simulink model "MSFartoystyring"  (R2016a)
settings: Solver=ode45  StartTime=tstart  StopTime=tstop  RelTol=1e-3
values from neighbouring files (symbols this model uses):
  c = 0    [run_task_2_2.m]
  d1 = 1.0163    [run_task_2_2.m]
  d2 = 2.4413e-05    [run_task_2_2.m]
  K_d = (2*zeta*w_n*T - 1)/K    (= 268.173334927)    [run_task_2_2.m]
  K_i = K_p*w_n/10    (= 0.176946727827)    [run_task_2_2.m]
  K_is = lambda^2    [run_task_2_2.m]
  K_p = w_n^2*T/K    (= 17.6946727827)    [run_task_2_2.m]
  K_ps = 2*lambda    [run_task_2_2.m]
  m = 365.2560    (= 365.256)    [run_task_2_2.m]
  psi0 = deg2rad(150)    [run_task_2_2.m]
  r0 = 0    [run_task_2_2.m]
  tsamp = 10    [run_task_2_2.m]
  v0 = [6.63 0]'    [run_task_2_2.m]
  w_n = 0.1    [run_task_2_2.m]
  w_ns = 0.01    [run_task_2_2.m]
  zeta = 0.8    [run_task_2_2.m]
  zeta_s = 1    [run_task_2_2.m]
undefined symbols (not defined in the file or in its folder): msfartoystyring, WP
undefined symbols (not defined in the file): p0
settings Model: ExtModeAutoUpdateStatusClock=off  Creator=christh  LastModifiedBy=fredr
settings DataIOCC: LimitDataPoints=on  SaveFormat=Array  SignalLoggingSaveFormat=ModelDataLogs
settings OptimizationCC: ExpressionDepthLimit=2147483647  InitFltsAndDblsToZero=on
settings DebuggingCC: UnderspecifiedInitializationDetection=Classic  MergeDetectMultiDrivingBlocksExec=none  SolverPrmCheckMsg=warning  FcnCallInpInsideContextMsg=UseLocalSettings  AllowSymbolicDim=off  StateNameClashWarn=warning
settings HardwareCC: ProdBitPerPointer=32  ProdLargestAtomicFloat=None  ProdIntDivRoundTo=Undefined  ProdEndianess=Unspecified  ProdWordSize=32  ProdHWDeviceType=32-bit Generic
settings ModelReferenceCC: PropagateSignalLabelsOutOfModel=off
settings GRTTargetCC: CombineOutputUpdateFcns=off  GRTInterface=on
settings ConfigComp: CovModelRefEnable=Off

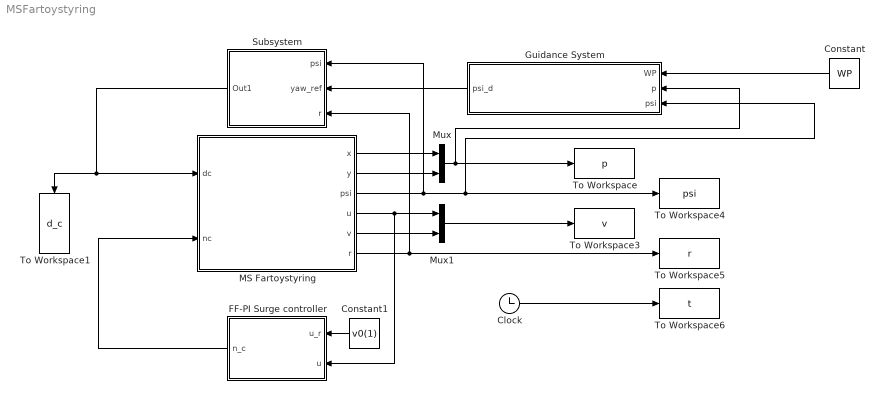
== system MSFartoystyring ==
  Clock : Clock
  Constant : Constant  Value=WP
  Constant1 : Constant  Value=v0(1)
  FF-PI Surge controller : Subsystem
  Guidance System : MATLAB Function  TreatAsAtomicUnit=on
  MS Fartoystyring : Subsystem  mask(MS Fartoystyring for Assignment 3 G&C){x0=p0(1), y0=p0(2), u0=v0(1), v0=v0(2), psi0=psi0, r0=r0, c=c}
      mask prompts: x0 "x(t0) (m)"; y0 "y(t0) (m)"; u0 "u(t0) (m/s)"; v0 "v(t0) (m/s)"; psi0 "psi(t0) (rad)"; r0 "r(t0) (rad/s)"; c "current (0 or 1)"
      mask help:
      | Block corresponding to Figure 1 in the assignment text. Gives the response of the ship.
      |
      | The design speed of MS Fartoystyring is u=8.23 m/s.
      |
      | Input:
      | dc: commanded rudder (rad), dmax=25*pi/180
      | nc: commanded shaft speed (rad/s), nmax=85*2*pi/60
      |
      | Output:
      | x: north pos (m)
      | y: east pos (m)
      | u: surge (m/s)
      | v: sway (m/s)
      | psi: heading (rad)
      | r: yaw (rad/s)
      mask Help: Comments, bugs and help requests can be directed to the TA. Email on course website.
  Mux : Mux  Inputs=2
  Mux1 : Mux  Inputs=2
  Subsystem : Subsystem
  To Workspace : ToWorkspace  VariableName=p  SampleTime=tsamp
  To Workspace1 : ToWorkspace  VariableName=d_c  SampleTime=tsamp
  To Workspace3 : ToWorkspace  VariableName=v  SampleTime=tsamp
  To Workspace4 : ToWorkspace  VariableName=psi  SampleTime=tsamp
  To Workspace5 : ToWorkspace  VariableName=r  SampleTime=tsamp
  To Workspace6 : ToWorkspace  VariableName=t  SampleTime=tsamp
  wires:
  Clock/1 -> To Workspace6/1
  MS Fartoystyring/1(x) -> Mux/1
  MS Fartoystyring/2(y) -> Mux/2
  MS Fartoystyring/4(u) -> FF-PI Surge controller/2(u), Mux1/1
  MS Fartoystyring/5(v) -> Mux1/2
  Mux/1 -> Guidance System/2(p), To Workspace/1
  Mux1/1 -> To Workspace3/1
  MS Fartoystyring/3(psi) -> Subsystem/1(psi), To Workspace4/1, Guidance System/3(psi)
  MS Fartoystyring/6(r) -> To Workspace5/1, Subsystem/3(r)
  FF-PI Surge controller/1(n_c) -> MS Fartoystyring/2(nc)
  Subsystem/1(Out1) -> To Workspace1/1, MS Fartoystyring/1(dc)
  Constant1/1 -> FF-PI Surge controller/1(u_r)
  Guidance System/1(psi_d) -> Subsystem/2(yaw_ref)
  Constant/1 -> Guidance System/1(WP)

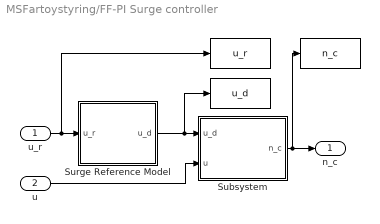
== system MSFartoystyring/FF-PI Surge controller ==
  u_r : Inport
  u : Inport  Port=2
  "      " : ToWorkspace  VariableName=u_d  SampleTime=tsamp
  " " : ToWorkspace  VariableName=n_c  SampleTime=tsamp
  "        " : ToWorkspace  VariableName=u_r  SampleTime=tsamp
  " Surge Reference Model" : Subsystem
  Subsystem : Subsystem
  n_c : Outport
  wires:
  u_r/1 -> " Surge Reference Model"/1(u_r), "        "/1
  " Surge Reference Model"/1(u_d) -> Subsystem/1(u_d), "      "/1
  u/1 -> Subsystem/2(u)
  Subsystem/1(n_c) -> " "/1, n_c/1

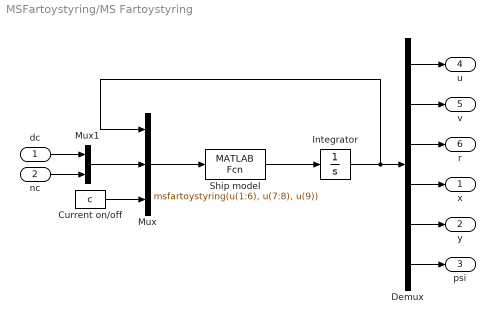
== system MSFartoystyring/MS Fartoystyring ==
  dc : Inport
  nc : Inport  Port=2
  Current on/off : Constant  Value=c
  Demux : Demux  Outputs=6
  Integrator : Integrator  InitialCondition=[u0 v0 r0 x0 y0 psi0]'
  Mux : Mux  Inputs=3
  Mux1 : Mux  Inputs=2
  Ship model : MATLABFcn  MATLABFcn=msfartoystyring(u(1:6), u(7:8), u(9))  OutputDimensions=6
  x : Outport
  y : Outport  Port=2
  psi : Outport  Port=3
  u : Outport  Port=4
  v : Outport  Port=5
  r : Outport  Port=6
  wires:
  Integrator/1 -> Mux/1, Demux/1
  Mux1/1 -> Mux/2
  dc/1 -> Mux1/1
  nc/1 -> Mux1/2
  Demux/1 -> u/1
  Demux/2 -> v/1
  Demux/3 -> r/1
  Demux/4 -> x/1
  Demux/5 -> y/1
  Demux/6 -> psi/1
  Current on/off/1 -> Mux/3
  Ship model/1 -> Integrator/1
  Mux/1 -> Ship model/1

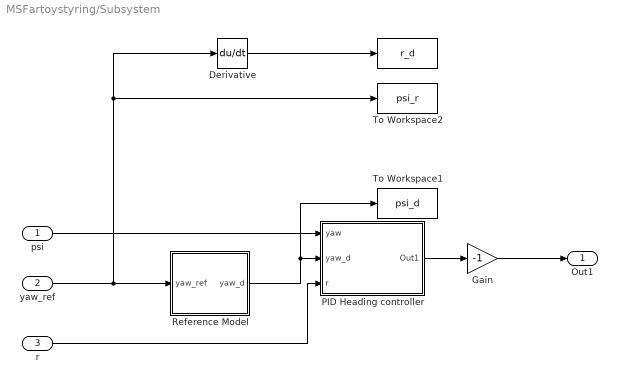
== system MSFartoystyring/Subsystem ==
  psi : Inport
  yaw_ref : Inport  Port=2
  r : Inport  Port=3
  " " : ToWorkspace  VariableName=r_d  SampleTime=tsamp
  Derivative : Derivative
  Gain : Gain  Gain=-1
  PID Heading controller : Subsystem
  Reference Model : Subsystem
  To Workspace1 : ToWorkspace  VariableName=psi_d  SampleTime=tsamp
  To Workspace2 : ToWorkspace  VariableName=psi_r  SampleTime=tsamp
  Out1 : Outport
  wires:
  r/1 -> PID Heading controller/3(r)
  Reference Model/1(yaw_d) -> PID Heading controller/2(yaw_d), To Workspace1/1
  yaw_ref/1 -> Reference Model/1(yaw_ref), To Workspace2/1, Derivative/1
  PID Heading controller/1(Out1) -> Gain/1
  Gain/1 -> Out1/1
  Derivative/1 -> " "/1
  psi/1 -> PID Heading controller/1(yaw)

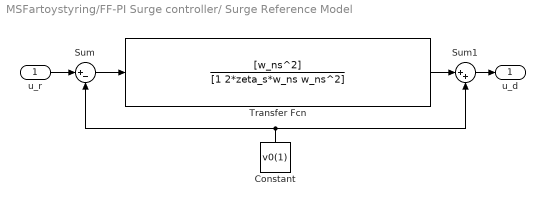
== system MSFartoystyring/FF-PI Surge controller/ Surge Reference Model ==
  u_r : Inport
  Constant : Constant  Value=v0(1)
  Sum : Sum  Inputs=|+-
  Sum1 : Sum  Inputs=|++
  Transfer Fcn : TransferFcn  Numerator=[w_ns^2]  Denominator=[1 2*zeta_s*w_ns w_ns^2]
  u_d : Outport
  wires:
  u_r/1 -> Sum/1
  Sum/1 -> Transfer Fcn/1
  Sum1/1 -> u_d/1
  Transfer Fcn/1 -> Sum1/1
  Constant/1 -> Sum1/2, Sum/2

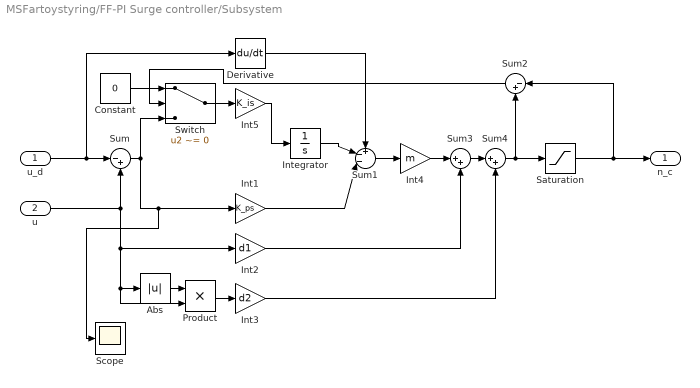
== system MSFartoystyring/FF-PI Surge controller/Subsystem ==
  u_d : Inport
  u : Inport  Port=2
  Abs : Abs
  Constant : Constant  Value=0
  Derivative : Derivative
  Int1 : Gain  Gain=K_ps
  Int2 : Gain  Gain=d1
  Int3 : Gain  Gain=d2
  Int4 : Gain  Gain=m
  Int5 : Gain  Gain=K_is
  Integrator : Integrator
  Product : Product
  Saturation : Saturate  UpperLimit=85*2*pi/60  LowerLimit=-85*2*pi/60  ZeroCross=off
  Scope : Scope
  Sum : Sum  Inputs=|-+
  Sum1 : Sum  Inputs=+--|
  Sum2 : Sum  Inputs=|-+
  Sum3 : Sum  Inputs=|++
  Sum4 : Sum  Inputs=|++
  Switch : Switch  Criteria=u2 ~= 0  ZeroCross=off
  n_c : Outport
  wires:
  Switch/1 -> Int5/1
  Int1/1 -> Sum1/3
  Int4/1 -> Sum3/1
  Sum3/1 -> Sum4/1
  Int3/1 -> Sum4/2
  u/1 -> Sum/2, Int2/1, Abs/1, Product/2
  Sum4/1 -> Sum2/2, Saturation/1
  u_d/1 -> Derivative/1, Sum/1
  Constant/1 -> Switch/1
  Sum2/1 -> Switch/2
  Sum/1 -> Switch/3, Scope/1, Int1/1
  Derivative/1 -> Sum1/1
  Integrator/1 -> Sum1/2
  Saturation/1 -> n_c/1, Sum2/1
  Int2/1 -> Sum3/2
  Product/1 -> Int3/1
  Sum1/1 -> Int4/1
  Int5/1 -> Integrator/1
  Abs/1 -> Product/1

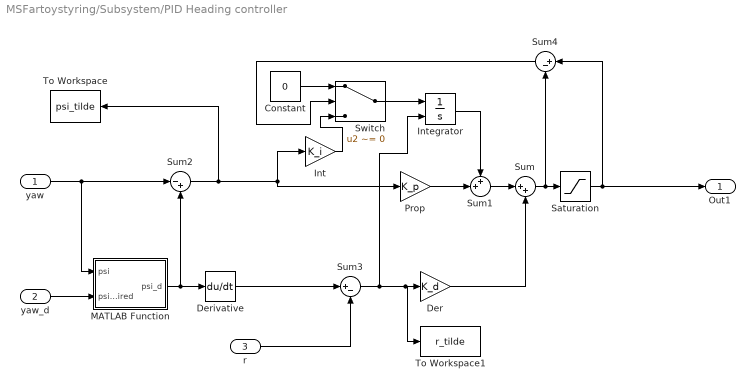
== system MSFartoystyring/Subsystem/PID Heading controller ==
  yaw : Inport
  yaw_d : Inport  Port=2
  r : Inport  Port=3
  Constant : Constant  Value=0
  Der : Gain  Gain=K_d
  Derivative : Derivative
  Int : Gain  Gain=K_i
  Integrator : Integrator  ExternalReset=either
  MATLAB Function : MATLAB Function  TreatAsAtomicUnit=on
  Prop : Gain  Gain=K_p
  Saturation : Saturate
  Sum : Sum  Inputs=|++
  Sum1 : Sum  Inputs=++|
  Sum2 : Sum  Inputs=|-+
  Sum3 : Sum  Inputs=|+-
  Sum4 : Sum  Inputs=|+-
  Switch : Switch  Criteria=u2 ~= 0
  To Workspace : ToWorkspace  VariableName=psi_tilde  SampleTime=tsamp
  To Workspace1 : ToWorkspace  VariableName=r_tilde  SampleTime=tsamp
  Out1 : Outport
  wires:
  Der/1 -> Sum/2
  Sum/1 -> Sum4/2, Saturation/1
  Sum1/1 -> Sum/1
  yaw/1 -> MATLAB Function/1(psi), Sum2/1
  yaw_d/1 -> MATLAB Function/2(psi_desired)
  Derivative/1 -> Sum3/1
  Sum3/1 -> Integrator/2, To Workspace1/1, Der/1
  r/1 -> Sum3/2
  Saturation/1 -> Sum4/1, Out1/1
  Integrator/1 -> Sum1/1
  Prop/1 -> Sum1/2
  Switch/1 -> Integrator/1
  Int/1 -> Switch/3
  Constant/1 -> Switch/1
  Sum4/1 -> Switch/2
  Sum2/1 -> Prop/1, Int/1, To Workspace/1
  MATLAB Function/1(psi_d) -> Sum2/2, Derivative/1

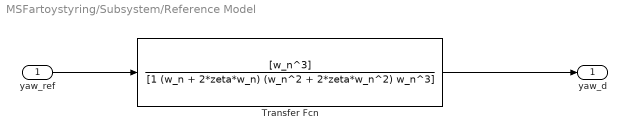
== system MSFartoystyring/Subsystem/Reference Model ==
  yaw_ref : Inport
  Transfer Fcn : TransferFcn  Numerator=[w_n^3]  Denominator=[1 (w_n + 2*zeta*w_n) (w_n^2 + 2*zeta*w_n^2) w_n^3]
  yaw_d : Outport
  wires:
  Transfer Fcn/1 -> yaw_d/1
  yaw_ref/1 -> Transfer Fcn/1

== matlab function MSFartoystyring/Subsystem/PID Heading controller/MATLAB Function ==
  data: psi input; psi_d output; psi_desired input
function psi_d = fcn(psi,psi_desired)

% The relative error shall never be higher than +/-180 degrees

psi_pi = mod(psi+pi,2*pi)-pi;                  % Map 2 +/-pi
psi_tilde = psi_desired-psi_pi;                % Angle difference [-2pi,pi]
psi_tilde = mod(psi_tilde+pi,2*pi)-pi;         % Map 2 +/-pi

psi_d = psi+psi_tilde;

== matlab function MSFartoystyring/Guidance System ==
  data: WP input; p input; psi input; psi_d output
function psi_d  = guidancesystem(WP, p, psi )
%GUIDANCESYSTEM A LOS based guidance system

% Keep track of current waypoint
persistent k;

% Acceptance circle radius
Lpp = 304.8;
R = 2*Lpp;

if isempty(k)
    k = 1; % Set next waypoint to first one. Current is init pos
end
   
% Extract current waypoint and next.
xn = WP(1,k+1); % next WP x-pos
yn = WP(2,k+1); % next WP y-post

xk = WP(1,k); % Current WP x-pos
yk = WP(2,k); % Current WP y-pos

% Extract current position.
x = p(1);
y = p(2);

% Check if we can switch to next waypoint
if ( ((xn - x)^2 + (yn - y)^2 <= R^2) && k < length(WP))
    k = k + 1;
    % Update waypoints
    xk = xn;
    yk = yn;
    
    xn = WP(1,k+1);
    yn = WP(2,k+1);
end

% Compute the path tangential angle
alpha = atan2(yn - yk, xn - xk);

Rp = [cos(alpha) -sin(alpha);
      sin(alpha) cos(alpha)];
  
% Distance from craft to current waypoint
p = p - WP(:,k);

% Position of craft in path-fixed ref frame
eps = Rp'*p;

s = eps(1);
e = eps(2);

% Compute the inverse error gain
delta = sqrt(max(0.01, R^2-e^2));

% Compute the desired heading
psi_d = alpha + atan2(-e,delta); % Will be in range  -pi, pi

end
